simulink model "AVR_H_inf_LMI__"  (R2022a)
settings: Solver=VariableStepAuto  StartTime=0.0  StopTime=300  RelTol=1e-3
libraries: simulink x1
settings Model: Creator=asus  LastModifiedBy=asus

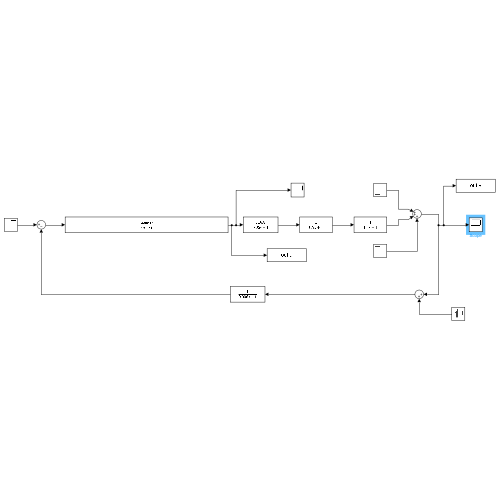
[thumbnail: Simulink's stored preview of the top-level diagram]
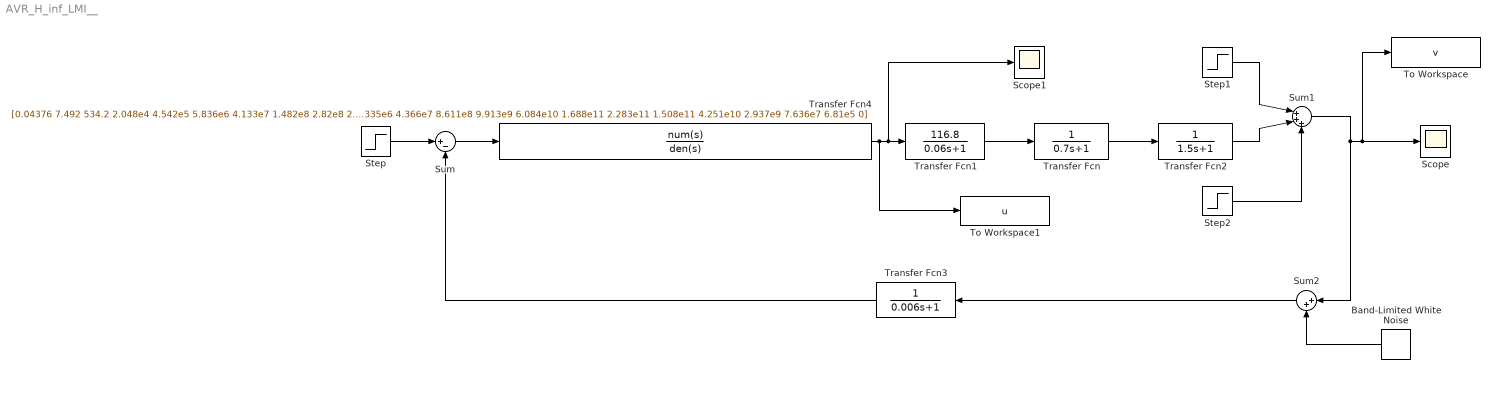
== system AVR_H_inf_LMI__ ==
  Band-Limited White Noise : simulink/Sources/Band-Limited White Noise  Cov=[0]  Ts=0.1  seed=[23341]
  Scope : Scope
  Scope1 : Scope
  Step : Step  Time=0  SampleTime=0
  Step1 : Step  Time=100  SampleTime=0
  Step2 : Step  Time=200  After=-1  SampleTime=0
  Sum : Sum  Inputs=|+-
  Sum1 : Sum  Inputs=|+++
  Sum2 : Sum  Inputs=|++
  To Workspace : ToWorkspace  VariableName=v  SaveFormat=Timeseries  SampleTime=-1
  To Workspace1 : ToWorkspace  VariableName=u  SaveFormat=Timeseries  SampleTime=-1
  Transfer Fcn : TransferFcn  Denominator=[0.7 1]
  Transfer Fcn1 : TransferFcn  Numerator=[116.8]  Denominator=[0.06 1]
  Transfer Fcn2 : TransferFcn  Denominator=[1.5 1]
  Transfer Fcn3 : TransferFcn  Denominator=[0.006 1]
  Transfer Fcn4 : TransferFcn  Numerator=[0.04376 7.492 534.2 2.048e4 4.542e5 5.836e6 4.133e7 1.482e8 2.82e8 2.905e8 1.552e8 3.685e7 2.257e6 5.292e4 430.3]  Denominator=[1 240.1 2.423e4 1.335e6 4.366e7 8.611e8 9.913e9 6.084e10 1.688e11 2.283e11 1.508e11 4.251e10 2.937e9 7.636e7 6.81e5 0]
  wires:
  Band-Limited White Noise/1 -> Sum2/2
  Transfer Fcn1/1 -> Transfer Fcn/1
  Sum2/1 -> Transfer Fcn3/1
  Step1/1 -> Sum1/1
  Step2/1 -> Sum1/3
  Sum1/1 -> Sum2/1, To Workspace/1, Scope/1
  Step/1 -> Sum/1
  Transfer Fcn2/1 -> Sum1/2
  Transfer Fcn/1 -> Transfer Fcn2/1
  Sum/1 -> Transfer Fcn4/1
  Transfer Fcn4/1 -> To Workspace1/1, Scope1/1, Transfer Fcn1/1
  Transfer Fcn3/1 -> Sum/2
